simulink model "sdruqpsktx_BPSK"  (R2020a)
settings: Solver=FixedStepDiscrete  StartTime=0.0  StopTime=inf  RelTol=1e-3
PreLoadFcn:
  | platform = sdruExampleFindRadio;
  | sdrqpsktx = sdruqpsktransmitter_init(platform, false);
  | 
  | clear platform
PostLoadFcn:
  | sdruExampleSetAvailableRadio;
InitFcn:
  | platform = get_param([gcs '/USRP Transmitter'], 'Platform');
  | sdrqpsktx = sdruqpsktransmitter_init(platform, false);
  | switch platform
  |   case 'N300'
  |     set_param([gcs,'/USRP Transmitter'], 'masterClkRateN300','153.6e6');
  |   case 'N310'
  |     set_param([gcs,'/USRP Transmitter'], 'masterClkRateN310','153.6e6');
  | end
  | clear platform
libraries: commdigbbndpm3 x2, dspsigops x1, commsequence2 x1, dspsrcs4 x1, sdrublksprivate x1, commfilt2 x1, commsdrhw_v2 x1
settings Model: FPTRunName=Active  SimulationMode=accelerator  Creator=The MathWorks, Inc.  LastModifiedBy=peytonaplin
settings DataIOCC: LimitDataPoints=on  SaveFormat=Array  SaveOutput=off  SaveTime=off  ReturnWorkspaceOutputs=off
settings OptimizationCC: BooleanDataType=off  DefaultParameterBehavior=Inlined  ExpressionDepthLimit=2147483647  LocalBlockOutputs=off  LifeSpan=inf
settings DebuggingCC: AlgebraicLoopMsg=error  UnderspecifiedInitializationDetection=Classic  MergeDetectMultiDrivingBlocksExec=none  SolverPrmCheckMsg=warning  SingleTaskRateTransMsg=error  FcnCallInpInsideContextMsg=warning  AllowSymbolicDim=off  StateNameClashWarn=warning  SFUnexpectedBacktrackingDiag=warning  SFNoUnconditionalDefaultTransitionDiag=warning  SFExecutionAtInitializationDiag=none  ArithmeticOperatorsInVariantConditions=warning
settings HardwareCC: ProdBitPerPointer=32  ProdBitPerSizeT=32  ProdBitPerPtrDiffT=32  ProdLargestAtomicFloat=None  ProdIntDivRoundTo=Undefined  ProdEndianess=Unspecified  ProdWordSize=32  ProdHWDeviceType=32-bit Generic  TargetBitPerPointer=64  TargetBitPerSizeT=64  TargetBitPerPtrDiffT=64  TargetLongLongMode=on  TargetIntDivRoundTo=Zero  TargetEndianess=LittleEndian  TargetWordSize=64  TargetHWDeviceType=Generic->MATLAB Host Computer  ProdEqTarget=off
settings ModelReferenceCC: PropagateSignalLabelsOutOfModel=off
settings SFSimCC: SimUseLocalCustomCode=off  CustomCodeUndefinedFunction=UseInterfaceOnly
settings RTWCC: RTWUseLocalCustomCode=off
settings RTWCC: CustomSourceCode=|
  | #include <stdio.h>
  | #include <stdlib.h>
settings CodeAppCC: StateflowObjectComments=on
settings GRTTargetCC: TargetLangStandard=C89/C90 (ANSI)  CombineOutputUpdateFcns=off  GRTInterface=on
settings ConfigComp: CovMetricSettings=dw  CovHtmlReporting=on  CovSaveCumulativeToWorkspaceVar=on  CovSaveSingleToWorkspaceVar=on  CovExternalEMLEnable=off  CovSFcnEnable=off

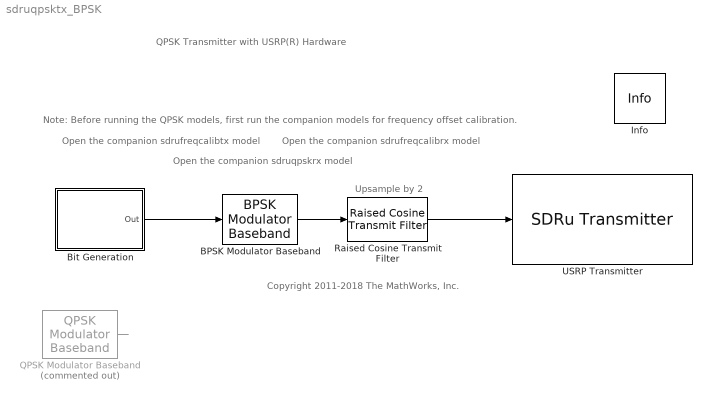
== system sdruqpsktx_BPSK ==
  note: Upsample by 2
  note: QPSK Transmitter with USRP(R) Hardware
  note: Open the companion sdruqpskrx model
  note: Note: Before running the QPSK models, first run the companion models for frequency offset calibration.
  note: Open the companion sdrufreqcalibrx model
  note: Open the companion sdrufreqcalibtx model
  note: Copyright 2011-2018 The MathWorks, Inc.
  BPSK Modulator Baseband : commdigbbndpm3/BPSK Modulator Baseband  Ph=0  outDtype=double  outWordLen=16  outUDDataType=sfix(16)  outFracLenMode=Best precision  outFracLen=15  outDataTypeStr=double  outLastDataTypeStr=double
  Bit Generation : Subsystem
      mask Display: disp('Bits Generation')
  Info : sdrublksprivate/Info  SystemSampleTime=-1  Latency=0  AutoFrameSizeCalculation=off
      settings: SourceProductBaseCode=USRP
  QPSK Modulator Baseband : commdigbbndpm3/QPSK Modulator Baseband  Commented=on  InType=Bit  Enc=Gray  Ph=pi/4  outDtype=double  outWordLen=16  outUDDataType=sfix(16)  outFracLenMode=Best precision  outFracLen=15  outDataTypeStr=double  outLastDataTypeStr=double
  Raised Cosine Transmit Filter : commfilt2/Raised Cosine Transmit Filter  filtType=Square root  R=sdrqpsktx.RolloffFactor  filtSpan=sdrqpsktx.RaisedCosineFilterSpan  N=sdrqpsktx.Interpolation  filterGain=1  InputProcessing=Columns as channels (frame based)  RateOptions=Enforce single-rate processing  framing=Mute  checkCoeff=off  variableName=rcTxFilt1  checkGain=Normalized  sampMode=Mute  saveAsFlag=0  currentFiltSpan=10  D=5  launchFVT=on  roundingMode=Floor  overflowMode=off  coeffDataTypeStr=Inherit: Same word length as input  coeffMin=[]  coeffMax=[]  coeffLastDataTypeStr=Inherit: Same word length as input  outputDataTypeStr=Inherit: Same as accumulator  outputMin=[]  outputMax=[]  outputLastDataTypeStr=Inherit: Same as accumulator
  USRP Transmitter : commsdrhw_v2/SDRu Transmitter  rxtx=tx  initializeIPAddress=0  devMap=0  USRP2_IP=192.168.10.2  USRP_IP_X300=192.168.10.2  USRP_IP_X310=192.168.30.2  USRP_IP_N300=192.168.10.2  USRP_IP_N310=192.168.10.2  USRP_IP_N320=No devices found  USRP_serialNumB200=30B2ACA  USRP_serialNumB210=ECR04ZDBT  platform=N200/N210/USRP2  prevPlatform=N200/N210/USRP2  lastIPAddressPopup=192.168.10.2  USRP_ID=192.168.10.2  LastIPAddress=192.168.10.2  ChannelMapping=1  centerFrequencySrc=Dialog  centerFrequency=sdrqpsktx.USRPCenterFrequency  loOffsetSrc=Dialog  loOffset=0  gainSrc=Dialog  gain=sdrqpsktx.USRPGain  PPSSource=Internal  clockSource=Internal  masterClkRateParam=100e6  masterClkRateB200=sdrqpsktx.MasterClockRate  masterClkRateB210=sdrqpsktx.MasterClockRate  masterClkRateX300=200e6  masterClkRateX310=200e6  masterClkRateN300=153.6e6  masterClkRateN310=153.6e6  masterClkRateN320=200e6  decimInterpSrc=Dialog  lastDecimSource=Dialog  decimInterp=sdrqpsktx.USRPInterpolationFactor  USRP2_IP_NUM=[49 57 50 46 49 54 56 46 49 48 46 50]  frameLength=362  sampleRate=400000  TransportDataType=int16  outputDatatype=Same as transport data type  overrunUnderrunPort=off  sampleTime=1  dboardInfo=|  HOST_DATA_PORT=30000  HOST_CONTROL_PORT=30001  USRP2_DATA_PORT=32769  USRP2_CONTROL_PORT=32768  bufferMode=Continuous streaming  EnableBurstMode=off  NumFramesInBurst=100
      | dbid: 0
      |           dbName: 'no db found'
      |          freqMin: 0
      |          freqMax: 0
      |          gainMin: 0
      |          gainMax: 0
      |     gainStepSize: 0
      settings: SourceProductBaseCode=USRP
  wires:
  Bit Generation/1(Out) -> BPSK Modulator Baseband/1
  QPSK Modulator Baseband/1 -> ?
  Raised Cosine Transmit Filter/1 -> USRP Transmitter/1
  BPSK Modulator Baseband/1 -> Raised Cosine Transmit Filter/1

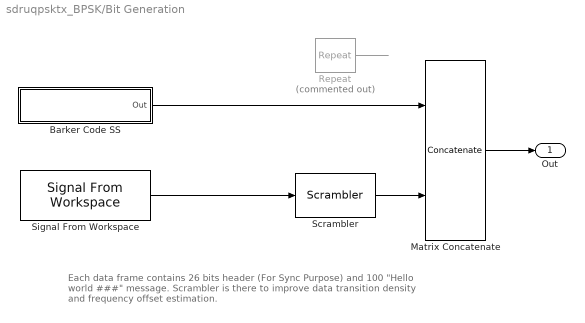
== system sdruqpsktx_BPSK/Bit Generation ==
  note: Each data frame contains 26 bits header (For Sync Purpose) and 100
      | "Hello world ###" message. Scrambler is there to improve data
      | transition density and frequency offset estimation.
  Barker Code SS : Subsystem
      mask Display: disp('Unipolar\nBarker Code')
  Matrix Concatenate : Concatenate  Mode=Multidimensional array
  Repeat : dspsigops/Repeat  Commented=on  N=2  InputProcessing=Columns as channels (frame based)  RateOptions=Enforce single-rate processing  ic=0  mode=Unused parameter value
  Scrambler : commsequence2/Scrambler  M=2  poly=[1 1 1 0 1]  iniStaSource=Dialog Parameter  ini_sta=[0 0 0 0]  resetViaPort=off
      settings: SourceProductBaseCode=CM
  Signal From Workspace : dspsrcs4/Signal From Workspace  X=sdrqpsktx.MessageBits  Ts=1/sdrqpsktx.PayloadLength*sdrqpsktx.FrameTime  nsamps=sdrqpsktx.MessageLength * 7 * sdrqpsktx.NumberOfMessage  OutputAfterFinalValue=Cyclic repetition  ignoreOrWarnInputAndFrameLengths=off  OutputFrames=off
  Out : Outport  VectorParamsAs1DForOutWhenUnconnected=off
  wires:
  Barker Code SS/1(Out) -> Matrix Concatenate/1
  Matrix Concatenate/1 -> Out/1
  Repeat/1 -> ?
  Scrambler/1 -> Matrix Concatenate/2
  Signal From Workspace/1 -> Scrambler/1

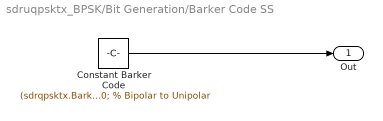
== system sdruqpsktx_BPSK/Bit Generation/Barker Code SS ==
  Constant Barker Code : Constant  Value=(sdrqpsktx.BarkerCode)' > 0; % Bipolar to Unipolar  VectorParams1D=off  OutDataTypeStr=double
  Out : Outport  VectorParamsAs1DForOutWhenUnconnected=off
  wires:
  Constant Barker Code/1 -> Out/1
